simulink model "Wanchao_shuttlecock_1"  (Simulink 7.7)
settings: Solver=ode4  StartTime=0.0  StopTime=inf  FixedStep=sample_time  RelTol=1e-3
InitFcn:
  | sample_time=0.005;%0.004;%0.0025;%0.02;
  | DeltaT = 0.02;
  | g = 9.81;
  | H0 = g%0.3165;
  | Kl = 1;
  | 
  | Omega_r = 1.6;%for Horizontal reference
  | Zeta_r = 0.7; %for Horizontal reference
  | Omega = 1.8;%for Horizontal Control
  | Zeta = 0.5;    %for Horizontal Control
  | 
  | Omega_h_r = 2.5; %for vertical reference
  | Zeta_h_r = 0.8;  %for vertical reference
  | Omega_h = 2.7;    %for vertical control
  | Zeta_h = 0.8;         %for vertical control
  | PI=pi;
  | 
  | Mass = 1.1;
  | Acc_Max = 4;
  | Acc_Max_h = 4;
  | 
  | Max_RP = 60;
  | 
  | load MaoBi_Oct04_2_int.mat
  | MB_Interp.time = [];
settings Model: Creator=ttcl3  LastModifiedBy=Birdman
settings SolverCC: MaxConsecutiveMinStep=auto
settings DebuggingCC: MultiTaskRateTransMsg=warning
settings SFSimCC: SimParseCustomCode=off

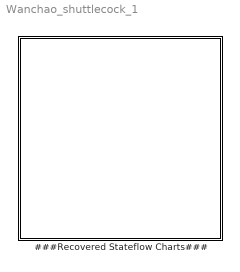
== system Wanchao_shuttlecock_1 ==
  ###Recovered Stateflow Charts### : Subsystem

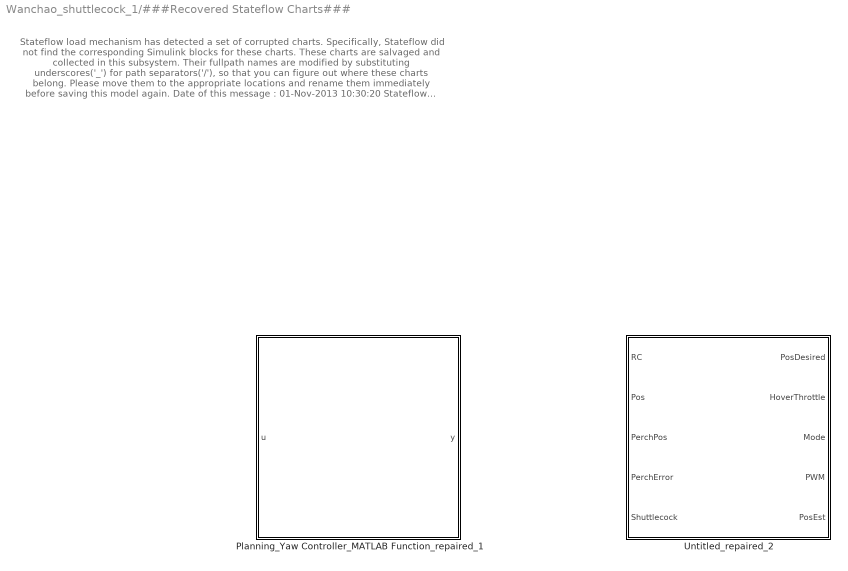
== system Wanchao_shuttlecock_1/###Recovered Stateflow Charts### ==
  note: Stateflow load mechanism has detected a set of corrupted charts.
      | Specifically, Stateflow did not find the corresponding Simulink blocks
      | for these charts. These charts are salvaged and collected in this subsystem.
      | Their fullpath names are modified by substituting underscores('_') for
      | path separators('/'), so that you can figure out where these charts belong.
      | Please move them to the appropriate locations and rename them immediately
      | before saving this model again.
      | Date of this message : 01-Nov-2013 10:30:20
      | Stateflow Version 7.5 (R2010a) dated Mar  4 2011, 22:36:02
  Planning_Yaw Controller_MATLAB Function_repaired_1 : Stateflow chart
  Untitled_repaired_2 : Stateflow chart

== matlab function ###Recovered Stateflow Charts###/Planning_Yaw Controller_MATLAB Function_repaired_1 ==
  data: u input double; y output double
function y = fcn(u)
%#codegen
y = u;
if y > pi    
    y = y - 2*pi;
elseif y < -pi
        y = y + 2*pi;
end

== stateflow chart ###Recovered Stateflow Charts###/Untitled_repaired_2 ==
  state Landing
    state Descending
      en:PosDesired = Pos;
      du:PosDesired[2] = (PerchPos[2]- PosDesired[2])*1*DeltaT + PosDesired[2] ;
    state CutThrottle
      du:HoverThrottle = (0 - HoverThrottle)*3*DeltaT + HoverThrottle ;
    (default) -> Descending
    Descending -> CutThrottle : [Pos[2] > (PerchPos[2]-0.1)]
  state Airborne
    state TakeOff
      du:HoverThrottle = (H0 - HoverThrottle)*3*DeltaT + HoverThrottle ;
    state Initialization
      du:PosDesired[0]=InitialPos[0];PosDesired[1]=InitialPos[1];
      PosDesired[2]=InitialPos[2];
    state SafyHover
      en:PosDesired = Pos; PosDesired[2]=-1.2;
    state Prelanding
      en:PosDesired[0]=InitialPos[0];PosDesired[1]=InitialPos[1];
      PosDesired[2]=InitialPos[2];
    state Descent
      en:PosDesired[2] = PerchPos[2]-0.15;
    state TrajE
      state DAQ
        en:i=0;
        du:PosShtlck[i]=Shuttlecock[0];PosShtlck[i+1]=Shuttlecock[1];
        PosShtlck[i+2]=Shuttlecock[2];PosShtlck[i+3]=Shuttlecock[3];
        PosShtlck[i+4]=Shuttlecock[4];PosShtlck[i+5]=Shuttlecock[5];i=i+6;
      state Estimation
        en:[pxe,pye,pze]=TrajEst(PosShtlck,H);
        du:PosDesired[0]=pxe;
        PosDesired[1]=pye;
        PosDesired[2]=pze;
      Estimation -> DAQ : [(Shuttlecock[2]-H<-0.4)|(Shuttlecock[5]<0)]{i=0;}
      DAQ -> Estimation : [i==30]
      (default) -> DAQ
    (default) -> TakeOff : {PosDesired = Pos;PosDesired[2] =-1.2;}
    Initialization -> SafyHover [order 2] : [RC[5] > 0]
    TakeOff -> Initialization : after(3,sec)
    SafyHover -> Prelanding : after(3, sec)
    Prelanding -> Descent : [PerchError < 0.01]
    Initialization -> TrajE [order 1] : [(abs(Shuttlecock[0])<1)&(Shuttlecock[1]<2.8)&(Shuttlecock[2]<H)]
    TrajE -> SafyHover : [(RC[5] > 0)]
  (default) -> Landing : {HoverThrottle = 0;}
  Airborne -> Landing : [RC[6] < -0.5]
  Landing -> Airborne : [RC[6] > 0.5]
  data: Shtck function_input double; xe function_output double; Hz function_input double; ye function_output double; ze function_output double; PosDesired output double size=4; HoverThrottle output double size=1; Mode output uint8 size=1; RC input double size=8; Pos input double size=4; PerchPos input double size=4; DeltaT parameter double size=1; H0 parameter double size=1; Kl parameter double size=1; VelCmd local double size=2 =0; PWM output double; PerchError input double; PI parameter double size=1; Shuttlecock input double size=6; InitialPos constant double size=3 =[0,-1,-1.2]; i local double =0; PosShtlck local double size=30; PosEst output double size=3; PosShtl local double size=30; H constant double =-1.3; pxe local double; pye local double; pze local double
  data H settings: description=Target Height
  events: trigger local EITHER_EDGE_EVENT
  function [xe,ye,ze]=TrajEst(Shtck,Hz):
    | function [xe,ye,ze]=TrajEst(Shtck,Hz)
    | 
    | px=[0 0 0 0 0];
    | py=[0 0 0 0 0];
    | pz=[0 0 0 0 0];
    | vx=[0 0 0 0 0];
    | 
    | for j=1:5
    |     px(j)=Shtck(j*6-5);
    |     py(j)=Shtck(j*6-4);
    |     pz(j)=Shtck(j*6-3);
    |     vx(j)=Shtck(j*6-2);
    | end
    | 
    | x0=px(1);
    | y0=py(1);
    | sgn=sign(mean(vx));
    | dx=sgn*0.01;
    | x=-1:0.02:1;
    | y=3:-0.01:-1.5;
    | 
    | tr_zx=polyval(polyfit(px,pz,2),x);
    | tr_zy=polyval(polyfit(py,pz,2),y);
    | 
    | [~,kx]=min(abs(tr_zx-Hz));
    | [~,ky]=min(abs(tr_zy-Hz));
    | 
    | xe=x(kx);
    | ye=y(ky);
    | ze=Hz-0.1;
